simulink model "test_adc_ctrl"  (Simulink 7.4)
settings: Solver=ode45  StartTime=0.0  StopTime=100  RelTol=1e-3
libraries: xbsIndex_r4 x148, xps_library x36, isi_correlator_lib x19, dspsigops x16, casper_library x8
(part 2 of 2)

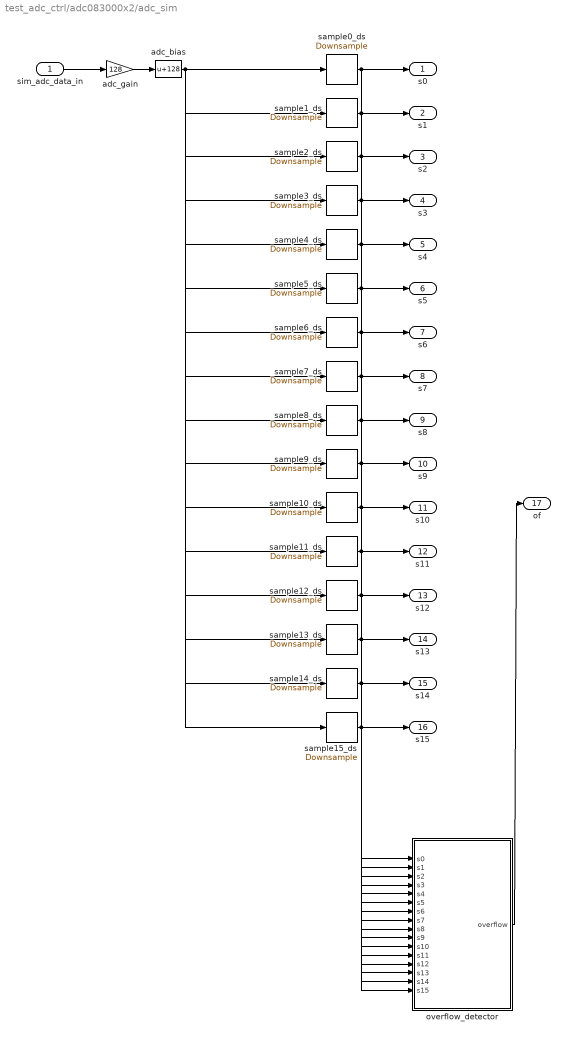
== system test_adc_ctrl/adc083000x2/adc_sim ==
  sim_adc_data_in : Inport  OutDataType=sfix(16)  OutScaling=2^0
  adc_bias : Bias  Bias=128  SaturateOnIntegerOverflow=on
  adc_gain : Gain  Gain=128  ParameterDataType=sfix(16)  ParameterScaling=2^0  OutDataType=sfix(16)  OutScaling=2^0
  overflow_detector : Subsystem  AncestorBlock=casper_library/Misc/of_detect_bus  mask(of_detect_bus){nStreams=16, bit_width=8}
      mask prompts: nStreams "Number of Streams"; bit_width "Bit Width"
      mask init:
      | adc_overflow_detector_init(gcb, ...
      |     'nStreams', nStreams, ...
      |     'bit_width', bit_width);
  sample0_ds : dspsigops/Downsample  N=16  phase=1  ic=0  smode=Force single rate  fmode=Maintain input frame size
  sample10_ds : dspsigops/Downsample  N=16  phase=11  ic=0  smode=Force single rate  fmode=Maintain input frame size
  sample11_ds : dspsigops/Downsample  N=16  phase=12  ic=0  smode=Force single rate  fmode=Maintain input frame size
  sample12_ds : dspsigops/Downsample  N=16  phase=13  ic=0  smode=Force single rate  fmode=Maintain input frame size
  sample13_ds : dspsigops/Downsample  N=16  phase=14  ic=0  smode=Force single rate  fmode=Maintain input frame size
  sample14_ds : dspsigops/Downsample  N=16  phase=15  ic=0  smode=Force single rate  fmode=Maintain input frame size
  sample15_ds : dspsigops/Downsample  N=16  phase=0  ic=0  smode=Force single rate  fmode=Maintain input frame size
  sample1_ds : dspsigops/Downsample  N=16  phase=2  ic=0  smode=Force single rate  fmode=Maintain input frame size
  sample2_ds : dspsigops/Downsample  N=16  phase=3  ic=0  smode=Force single rate  fmode=Maintain input frame size
  sample3_ds : dspsigops/Downsample  N=16  phase=4  ic=0  smode=Force single rate  fmode=Maintain input frame size
  sample4_ds : dspsigops/Downsample  N=16  phase=5  ic=0  smode=Force single rate  fmode=Maintain input frame size
  sample5_ds : dspsigops/Downsample  N=16  phase=6  ic=0  smode=Force single rate  fmode=Maintain input frame size
  sample6_ds : dspsigops/Downsample  N=16  phase=7  ic=0  smode=Force single rate  fmode=Maintain input frame size
  sample7_ds : dspsigops/Downsample  N=16  phase=8  ic=0  smode=Force single rate  fmode=Maintain input frame size
  sample8_ds : dspsigops/Downsample  N=16  phase=9  ic=0  smode=Force single rate  fmode=Maintain input frame size
  sample9_ds : dspsigops/Downsample  N=16  phase=10  ic=0  smode=Force single rate  fmode=Maintain input frame size
  s0 : Outport  OutDataType=sfix(16)  OutScaling=2^0
  s1 : Outport  Port=2  OutDataType=sfix(16)  OutScaling=2^0
  s2 : Outport  Port=3  OutDataType=sfix(16)  OutScaling=2^0
  s3 : Outport  Port=4  OutDataType=sfix(16)  OutScaling=2^0
  s4 : Outport  Port=5  OutDataType=sfix(16)  OutScaling=2^0
  s5 : Outport  Port=6  OutDataType=sfix(16)  OutScaling=2^0
  s6 : Outport  Port=7  OutDataType=sfix(16)  OutScaling=2^0
  s7 : Outport  Port=8  OutDataType=sfix(16)  OutScaling=2^0
  s8 : Outport  Port=9  OutDataType=fixdt(1, 16)  OutScaling=2^0
  s9 : Outport  Port=10  OutDataType=fixdt(1, 16)  OutScaling=2^0
  s10 : Outport  Port=11  OutDataType=fixdt(1, 16)  OutScaling=2^0
  s11 : Outport  Port=12  OutDataType=fixdt(1, 16)  OutScaling=2^0
  s12 : Outport  Port=13  OutDataType=fixdt(1, 16)  OutScaling=2^0
  s13 : Outport  Port=14  OutDataType=fixdt(1, 16)  OutScaling=2^0
  s14 : Outport  Port=15  OutDataType=fixdt(1, 16)  OutScaling=2^0
  s15 : Outport  Port=16  OutDataType=fixdt(1, 16)  OutScaling=2^0
  of : Outport  Port=17  OutDataType=sfix(16)  OutScaling=2^0
  wires:
  sim_adc_data_in/1 -> adc_gain/1
  adc_gain/1 -> adc_bias/1
  overflow_detector/1(overflow) -> of/1
  adc_bias/1 -> sample0_ds/1, sample1_ds/1, sample2_ds/1, sample3_ds/1, sample4_ds/1, sample5_ds/1, sample6_ds/1, sample7_ds/1, sample8_ds/1, sample9_ds/1, sample10_ds/1, sample11_ds/1, sample12_ds/1, sample13_ds/1, sample14_ds/1, sample15_ds/1
  sample0_ds/1 -> overflow_detector/1(s0), s0/1
  sample1_ds/1 -> overflow_detector/2(s1), s1/1
  sample2_ds/1 -> overflow_detector/3(s2), s2/1
  sample3_ds/1 -> overflow_detector/4(s3), s3/1
  sample4_ds/1 -> overflow_detector/5(s4), s4/1
  sample5_ds/1 -> overflow_detector/6(s5), s5/1
  sample6_ds/1 -> overflow_detector/7(s6), s6/1
  sample7_ds/1 -> overflow_detector/8(s7), s7/1
  sample8_ds/1 -> overflow_detector/9(s8), s8/1
  sample9_ds/1 -> overflow_detector/10(s9), s9/1
  sample10_ds/1 -> overflow_detector/11(s10), s10/1
  sample11_ds/1 -> overflow_detector/12(s11), s11/1
  sample12_ds/1 -> overflow_detector/13(s12), s12/1
  sample13_ds/1 -> overflow_detector/14(s13), s13/1
  sample14_ds/1 -> overflow_detector/15(s14), s14/1
  sample15_ds/1 -> overflow_detector/16(s15), s15/1

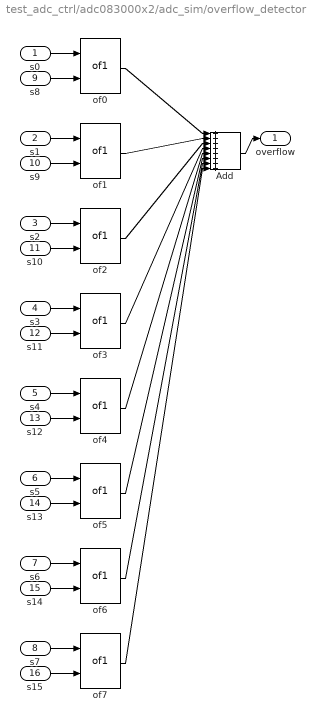
== system test_adc_ctrl/adc083000x2/adc_sim/overflow_detector ==
  s0 : Inport  OutDataType=fixdt(1, 16)  OutScaling=2^0
  s1 : Inport  Port=2  OutDataType=fixdt(1, 16)  OutScaling=2^0
  s2 : Inport  Port=3  OutDataType=fixdt(1, 16)  OutScaling=2^0
  s3 : Inport  Port=4  OutDataType=fixdt(1, 16)  OutScaling=2^0
  s4 : Inport  Port=5  OutDataType=fixdt(1, 16)  OutScaling=2^0
  s5 : Inport  Port=6  OutDataType=fixdt(1, 16)  OutScaling=2^0
  s6 : Inport  Port=7  OutDataType=fixdt(1, 16)  OutScaling=2^0
  s7 : Inport  Port=8  OutDataType=fixdt(1, 16)  OutScaling=2^0
  s8 : Inport  Port=9  OutDataType=fixdt(1, 16)  OutScaling=2^0
  s9 : Inport  Port=10  OutDataType=fixdt(1, 16)  OutScaling=2^0
  s10 : Inport  Port=11  OutDataType=fixdt(1, 16)  OutScaling=2^0
  s11 : Inport  Port=12  OutDataType=fixdt(1, 16)  OutScaling=2^0
  s12 : Inport  Port=13  OutDataType=fixdt(1, 16)  OutScaling=2^0
  s13 : Inport  Port=14  OutDataType=fixdt(1, 16)  OutScaling=2^0
  s14 : Inport  Port=15  OutDataType=fixdt(1, 16)  OutScaling=2^0
  s15 : Inport  Port=16  OutDataType=fixdt(1, 16)  OutScaling=2^0
  Add : Sum  Inputs=++++++++  OutDataType=fixdt(1, 16)  OutScaling=2^-10
  of{0..7} (8 alike) : casper_library/Misc/of1  SystemSampleTime=-1  bit_num=0  n_adc_bits=8
  overflow : Outport  OutDataType=fixdt(1, 16)  OutScaling=2^0
  wires:
  s0/1 -> of0/1
  s8/1 -> of0/2
  of0/1 -> Add/1
  s1/1 -> of1/1
  s9/1 -> of1/2
  of1/1 -> Add/2
  s2/1 -> of2/1
  s10/1 -> of2/2
  of2/1 -> Add/3
  s3/1 -> of3/1
  s11/1 -> of3/2
  of3/1 -> Add/4
  s4/1 -> of4/1
  s12/1 -> of4/2
  of4/1 -> Add/5
  s5/1 -> of5/1
  s13/1 -> of5/2
  of5/1 -> Add/6
  s6/1 -> of6/1
  s14/1 -> of6/2
  of6/1 -> Add/7
  s7/1 -> of7/1
  s15/1 -> of7/2
  of7/1 -> Add/8
  Add/1 -> overflow/1
